simulink model "vx_vy_parallel_dk_v2_3b2_compile_harness"  (R2024a)
settings: Solver=FixedStepDiscrete  StartTime=0  StopTime=0.1  FixedStep=0.001  RelTol=1e-3
model workspace (MAT data in the model file):
  vy_v17_mode_code = 20
undefined symbols (not defined in the file or in its folder): vy_dynamic_ekf_v1_17
libraries: simulink x2
settings Model: Creator=21180  LastModifiedBy=21180

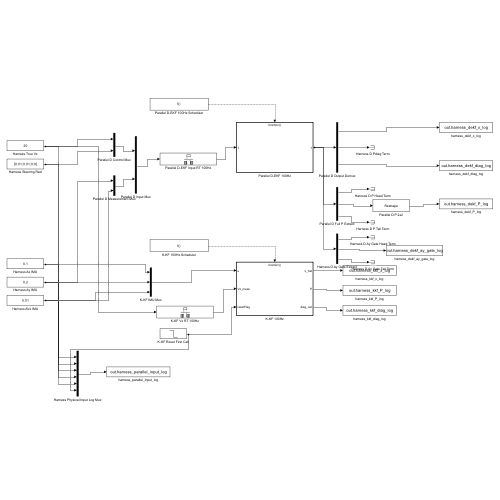
[thumbnail: Simulink's stored preview of the top-level diagram]
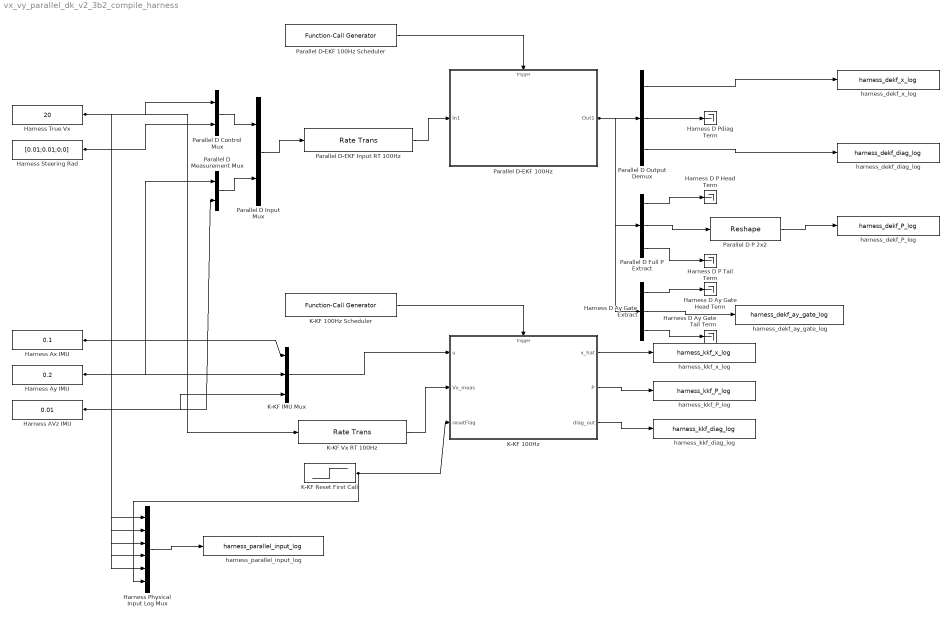
== system vx_vy_parallel_dk_v2_3b2_compile_harness ==
  Harness AVz IMU : Constant  Value=0.01  OutDataTypeStr=double  SampleTime=0.01
  Harness Ax IMU : Constant  Value=0.1  OutDataTypeStr=double  SampleTime=0.01
  Harness Ay IMU : Constant  Value=0.2  OutDataTypeStr=double  SampleTime=0.01
  Harness D Ay Gate Extract : Demux  Outputs=[59 1 9]
  Harness D Ay Gate Head Term : Terminator
  Harness D Ay Gate Tail Term : Terminator
  Harness D P Head Term : Terminator
  Harness D P Tail Term : Terminator
  Harness D Pdiag Term : Terminator
  Harness Physical Input Log Mux : Mux  Inputs=[1 1 1 1 4 1]
  Harness Steering Rad : Constant  Value=[0.01;0.01;0;0]  OutDataTypeStr=double  SampleTime=0.01
  Harness True Vx : Constant  Value=20  OutDataTypeStr=double  SampleTime=0.001
  K-KF 100Hz : Subsystem  TreatAsAtomicUnit=on
  K-KF 100Hz Scheduler : simulink/Ports & Subsystems/Function-Call Generator  sample_time=0.01  numberOfIterations=1  DisallowWideOutput=off
  K-KF IMU Mux : Mux  Inputs=3
  K-KF Reset First Call : Step  Time=0.01  Before=1  After=0  SampleTime=0.01
  K-KF Vx RT 100Hz : RateTransition  OutPortSampleTime=0.01
  Parallel D Control Mux : Mux  Inputs=[1 4]
  Parallel D Full P Extract : Demux  Outputs=[45 4 20]
  Parallel D Input Mux : Mux  Inputs=[5 2]
  Parallel D Measurement Mux : Mux  Inputs=2
  Parallel D Output Demux : Demux  Outputs=[2 2 65]
  Parallel D P 2x2 : Reshape  OutputDimensionality=Customize  OutputDimensions=[2 2]
  Parallel D-EKF 100Hz : Subsystem  TreatAsAtomicUnit=on
  Parallel D-EKF 100Hz Scheduler : simulink/Ports & Subsystems/Function-Call Generator  sample_time=0.01  numberOfIterations=1  DisallowWideOutput=off
  Parallel D-EKF Input RT 100Hz : RateTransition  OutPortSampleTime=0.01
  harness_dekf_P_log : ToWorkspace  VariableName=harness_dekf_P_log  SaveFormat=Timeseries  SampleTime=-1
  harness_dekf_ay_gate_log : ToWorkspace  VariableName=harness_dekf_ay_gate_log  SaveFormat=Timeseries  SampleTime=-1
  harness_dekf_diag_log : ToWorkspace  VariableName=harness_dekf_diag_log  SaveFormat=Timeseries  SampleTime=-1
  harness_dekf_x_log : ToWorkspace  VariableName=harness_dekf_x_log  SaveFormat=Timeseries  SampleTime=-1
  harness_kkf_P_log : ToWorkspace  VariableName=harness_kkf_P_log  SaveFormat=Timeseries  SampleTime=-1
  harness_kkf_diag_log : ToWorkspace  VariableName=harness_kkf_diag_log  SaveFormat=Timeseries  SampleTime=-1
  harness_kkf_x_log : ToWorkspace  VariableName=harness_kkf_x_log  SaveFormat=Timeseries  SampleTime=-1
  harness_parallel_input_log : ToWorkspace  VariableName=harness_parallel_input_log  SaveFormat=Timeseries  SampleTime=-1
  wires:
  Harness True Vx/1 -> Parallel D Control Mux/1, K-KF Vx RT 100Hz/1, Harness Physical Input Log Mux/4
  Harness Steering Rad/1 -> Parallel D Control Mux/2, Harness Physical Input Log Mux/5
  Harness Ay IMU/1 -> Parallel D Measurement Mux/1, K-KF IMU Mux/2, Harness Physical Input Log Mux/2
  Harness AVz IMU/1 -> Parallel D Measurement Mux/2, K-KF IMU Mux/3, Harness Physical Input Log Mux/3
  Parallel D Control Mux/1 -> Parallel D Input Mux/1
  Parallel D Measurement Mux/1 -> Parallel D Input Mux/2
  Parallel D Input Mux/1 -> Parallel D-EKF Input RT 100Hz/1
  Parallel D-EKF Input RT 100Hz/1 -> Parallel D-EKF 100Hz/1(In1)
  Parallel D-EKF 100Hz Scheduler/1 -> Parallel D-EKF 100Hz/Trigger
  Parallel D-EKF 100Hz/1(Out1) -> Parallel D Output Demux/1, Parallel D Full P Extract/1, Harness D Ay Gate Extract/1
  Parallel D Full P Extract/2 -> Parallel D P 2x2/1
  Harness Ax IMU/1 -> K-KF IMU Mux/1, Harness Physical Input Log Mux/1
  K-KF IMU Mux/1 -> K-KF 100Hz/1(u)
  K-KF Vx RT 100Hz/1 -> K-KF 100Hz/2(Vx_meas)
  K-KF Reset First Call/1 -> K-KF 100Hz/3(resetFlag), Harness Physical Input Log Mux/6
  K-KF 100Hz Scheduler/1 -> K-KF 100Hz/Trigger
  Parallel D Output Demux/1 -> harness_dekf_x_log/1
  Parallel D P 2x2/1 -> harness_dekf_P_log/1
  Parallel D Output Demux/3 -> harness_dekf_diag_log/1
  K-KF 100Hz/1(x_hat) -> harness_kkf_x_log/1
  K-KF 100Hz/2(P) -> harness_kkf_P_log/1
  K-KF 100Hz/3(diag_out) -> harness_kkf_diag_log/1
  Parallel D Output Demux/2 -> Harness D Pdiag Term/1
  Parallel D Full P Extract/1 -> Harness D P Head Term/1
  Parallel D Full P Extract/3 -> Harness D P Tail Term/1
  Harness D Ay Gate Extract/1 -> Harness D Ay Gate Head Term/1
  Harness D Ay Gate Extract/2 -> harness_dekf_ay_gate_log/1
  Harness D Ay Gate Extract/3 -> Harness D Ay Gate Tail Term/1
  Harness Physical Input Log Mux/1 -> harness_parallel_input_log/1

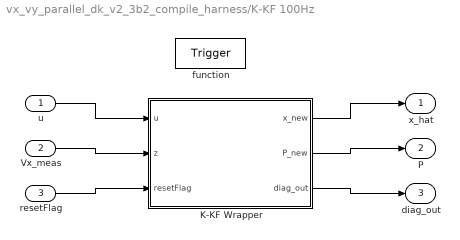
== system vx_vy_parallel_dk_v2_3b2_compile_harness/K-KF 100Hz ==
  u : Inport
  Vx_meas : Inport  Port=2
  resetFlag : Inport  Port=3
  function : TriggerPort  TriggerType=function-call  VariantControl=(inherit)
  K-KF Wrapper : MATLAB Function  TreatAsAtomicUnit=on
  x_hat : Outport
  P : Outport  Port=2
  diag_out : Outport  Port=3
  wires:
  K-KF Wrapper/3(diag_out) -> diag_out/1
  K-KF Wrapper/2(P_new) -> P/1
  K-KF Wrapper/1(x_new) -> x_hat/1
  resetFlag/1 -> K-KF Wrapper/3(resetFlag)
  Vx_meas/1 -> K-KF Wrapper/2(z)
  u/1 -> K-KF Wrapper/1(u)

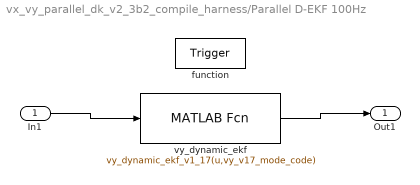
== system vx_vy_parallel_dk_v2_3b2_compile_harness/Parallel D-EKF 100Hz ==
  In1 : Inport
  function : TriggerPort  TriggerType=function-call  VariantControl=(inherit)
  vy_dynamic_ekf : MATLABFcn  MATLABFcn=vy_dynamic_ekf_v1_17(u,vy_v17_mode_code)  OutputDimensions=69
  Out1 : Outport
  wires:
  In1/1 -> vy_dynamic_ekf/1
  vy_dynamic_ekf/1 -> Out1/1

== matlab function vx_vy_parallel_dk_v2_3b2_compile_harness/K-KF 100Hz/K-KF Wrapper ==
  data: x_new output; u input; z input; resetFlag input; P_new output; diag_out output
function [x_new,P_new,diag_out] = kkf_wrapper(u,z,resetFlag)
%#codegen
[x_new,P_new,diag_out] = vy_kinematic_kf(u,z,resetFlag);
end
